simulink model "Lc_5_sim"  (R2022b)
settings: Solver=VariableStepAuto  StartTime=0.0  StopTime=10.0  RelTol=1e-3
settings Model: Creator=MSH8303  LastModifiedBy=MSH8303

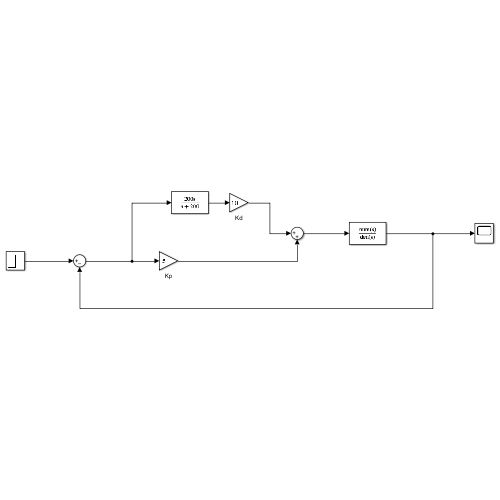
[thumbnail: Simulink's stored preview of the top-level diagram]
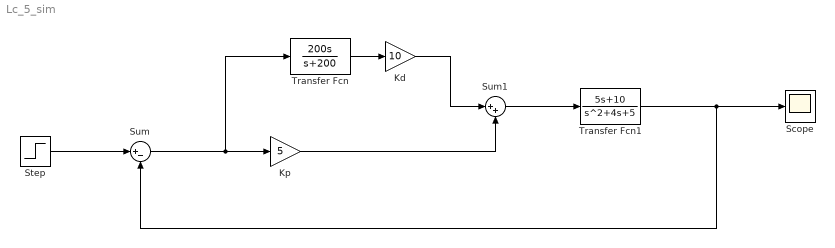
== system Lc_5_sim ==
  Kd : Gain  Gain=10
  Kp : Gain  Gain=5
  Scope : Scope
  Step : Step  SampleTime=0
  Sum : Sum  Inputs=|+-
  Sum1 : Sum  Inputs=|++
  Transfer Fcn : TransferFcn  Numerator=[200 0]  Denominator=[1 200]
  Transfer Fcn1 : TransferFcn  Numerator=[5 10]  Denominator=[1 4 5]
  wires:
  Step/1 -> Sum/1
  Sum/1 -> Transfer Fcn/1, Kp/1
  Transfer Fcn/1 -> Kd/1
  Kd/1 -> Sum1/1
  Kp/1 -> Sum1/2
  Sum1/1 -> Transfer Fcn1/1
  Transfer Fcn1/1 -> Sum/2, Scope/1
